simulink model "ROSFeedBackExample"  (R2019b)
settings: Solver=FixedStepDiscrete  StartTime=0.0  StopTime=Inf  FixedStep=0.02  RelTol=1e-3  EnableMultiTasking=on
values from neighbouring files (symbols this model uses):
  m = size(BW, 1)    [ClusterClean.m]    (also in ClusterFuck.m; dotDetection.m)
  X = (round((Ball{1,2}-571)*pixel2mm,2))    [ClusterClean.m]    (also in ClusterFuck.m = (round((Ball{1,2}-CueX)*pixel2mm+30-6.275,2)); PossibleShots.m = (round((balls{1,2})*pixel2mm,2)-6.71); dotDetection.m = rgb2lab(img))
  Y = (round((Ball{1,3}-41)*pixel2mm,2))    [ClusterClean.m]    (also in ClusterFuck.m = (round((Ball{1,3}-CueY)*pixel2mm+30,2)); PossibleShots.m = (round((balls{1,3})*pixel2mm,2)-6.71))
  Z = 80    [ClusterClean.m]    (also in ClusterFuck.m = 90; PossibleShots.m = 90)
undefined symbols (not defined in the file or in its folder): Angular, awayFromGoalThresh, Linear, loadingStation, logicalMap, objectPos, p, q0, refPos, tDuration, tStart, unloadingStations
libraries: sm_lib x153, nesl_utility x33, robotlib x7, robotmaniplib x5, simulink x3, robotalgslib x1
(part 1 of 4)
settings Model: Creator=The MathWorks, Inc.  LastModifiedBy=ryanl
settings DataIOCC: LimitDataPoints=on  SaveFormat=Array  ReturnWorkspaceOutputs=off
settings OptimizationCC: LifeSpan=Inf  MaxStackSize=64
settings DebuggingCC: SolverPrmCheckMsg=warning  AllowSymbolicDim=off  SFUnexpectedBacktrackingDiag=warning  SFNoUnconditionalDefaultTransitionDiag=warning  SFExecutionAtInitializationDiag=none  ArithmeticOperatorsInVariantConditions=warning
settings HardwareCC: ProdBitPerPointer=32  ProdBitPerSizeT=32  ProdBitPerPtrDiffT=32  ProdLargestAtomicFloat=None  ProdIntDivRoundTo=Undefined  ProdEndianess=Unspecified  ProdWordSize=32  ProdHWDeviceType=Generic->Unspecified (assume 32-bit Generic)  TargetHWDeviceType=Generic->Unspecified (assume 32-bit Generic)  UseEmbeddedCoderFeatures=off
settings ModelReferenceCC: PropagateSignalLabelsOutOfModel=off
settings SFSimCC: SimUseLocalCustomCode=off  CustomCodeUndefinedFunction=UseInterfaceOnly
settings RTWCC: SystemTargetFile=ert.tlc  HardwareBoard=Robot Operating System (ROS)  TemplateMakefile=ert_default_tmf  RTWUseLocalCustomCode=off  Toolchain=Catkin  TargetLang=C++
settings CodeAppCC: StateflowObjectComments=on
settings ERTTargetCC: MultiwordLength=2048  ERTCustomFileBanners=off  MultiInstanceERTCode=on  CodeInterfacePackaging=C++ class  SupportContinuousTime=on  SupportNonInlinedSFcns=on  RemoveResetFunc=off  SupportVariableSizeSignals=on  ModelStepFunctionPrototypeControlCompliant=off  RootIOFormat=Structure reference  ConvertIfToSwitch=off  SuppressUnreachableDefaultCases=off
settings ConfigComp: CovMetricSettings=dw  CovHtmlReporting=on  CovSaveCumulativeToWorkspaceVar=on  CovSaveSingleToWorkspaceVar=on  CovExternalEMLEnable=off  CovSFcnEnable=off

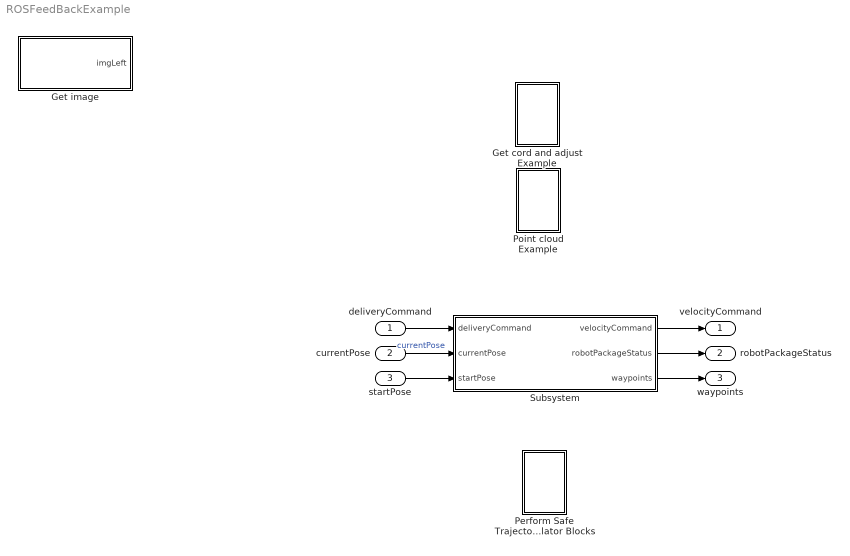
== system ROSFeedBackExample ==
  deliveryCommand : Inport  OutDataTypeStr=Bus: RobotDeliverCommand  BusOutputAsStruct=on
  currentPose : Inport  Port=2  PortDimensions=[3, 1]
  startPose : Inport  Port=3
  Get cord and adjust Example : Subsystem
  Get image : Subsystem
  Perform Safe Trajectory Tracking Control Using Robotics Manipulator Blocks : Subsystem
  Point cloud Example : Subsystem
  Subsystem : Subsystem
  velocityCommand : Outport
  robotPackageStatus : Outport  Port=2  OutDataTypeStr=Bus: RobotPackageStatus  BusOutputAsStruct=on
  waypoints : Outport  Port=3
  wires:
  deliveryCommand/1 -> Subsystem/1(deliveryCommand)
  currentPose/1 -> Subsystem/2(currentPose)  "currentPose"
  startPose/1 -> Subsystem/3(startPose)
  Subsystem/1(velocityCommand) -> velocityCommand/1
  Subsystem/2(robotPackageStatus) -> robotPackageStatus/1
  Subsystem/3(waypoints) -> waypoints/1

== system ROSFeedBackExample/Get cord and adjust Example ==
  note: The /odom topic represents orientation as a quarternion, so convert it to a yaw angle
  note: The desired (X,Y) position of the robot
      | (Colored blocks indicate tunable parameters)
  note: Feedback Control of a ROS-enabled Robot
  note: Copyright 2014-2016 The MathWorks, Inc.
  Bus Selector3 : BusSelector  OutputSignals=Pose.Pose.Position.X,Pose.Pose.Position.Y,Pose.Pose.Orientation.X,Pose.Pose.Orientation.Y,Pose.Pose.Orientation.Z,Pose.Pose.Orientation.W
  Command Velocity Publisher : Subsystem
  Conversion : MATLAB Function  TreatAsAtomicUnit=on
  Desired Position : Constant  Value=[-10 10]
  More Info : Subsystem
      settings: OpenFcn=showdemo(bdroot(gcb))
      mask Display: disp('?')
  Proportional Controller : Subsystem
  Scope : Scope
  Simulation Rate Control : MATLABSystem  System=ExampleHelperSimulationRateControl  SampleTime=0.02
      mask Type: ExampleHelperSimulationRateControl
      mask Display: disp('Rate Control');
  Subscribe : robotlib/Subscribe  topicSource=Select from ROS network  topic=/odom  messageType=nav_msgs/Odometry  sampleTime=-1  messageQueueLength=51
      settings: SourceProductName=ROS Toolbox
  wires:
  Bus Selector3/1 -> Proportional Controller/2(Position X)  "<X>"
  Subscribe/2 -> Bus Selector3/1
  Proportional Controller/1(Linear Velocity (v)) -> Command Velocity Publisher/1(v)
  Conversion/1(yaw) -> Proportional Controller/4(Orientation (theta))
  Desired Position/1 -> Proportional Controller/1(Desired position)
  Bus Selector3/2 -> Proportional Controller/3(Position Y)  "<Y>"
  Bus Selector3/3 -> Conversion/1(x)  "<X>"
  Bus Selector3/5 -> Conversion/3(z)  "<Z>"
  Subscribe/1 -> Command Velocity Publisher/Enable, Scope/1, Proportional Controller/Enable  "IsNew"
  Bus Selector3/4 -> Conversion/2(y)  "<Y>"
  Bus Selector3/6 -> Conversion/4(w)  "<W>"
  Proportional Controller/2(Angular Velocity (w)) -> Command Velocity Publisher/2(w)

== system ROSFeedBackExample/Get image ==
  note: Get Image AND Display
  Error Code Output : Display
  New Message : Display
  Read Image : robotlib/Read Image  MaximumImageSize=[480, 640]  ImageEncoding=rgb8  ShowAlphaOutput=off  ShowErrorCodeOutput=on  VariableSizeOutputs=off
      settings: SourceProductName=ROS Toolbox  SourceProductBaseCode=RR
  Video Viewer1 : VideoViewer  FigPos=[515 695 646 522]
  imgLeftSubscriber : robotlib/Subscribe  topicSource=Select from ROS network  topic=/image_test  messageType=sensor_msgs/Image  sampleTime=-1  messageQueueLength=1
      settings: SourceProductName=ROS Toolbox
  imgLeft : Outport
  wires:
  imgLeftSubscriber/2 -> Read Image/1
  Read Image/1 -> imgLeft/1, Video Viewer1/1
  Read Image/2 -> Error Code Output/1
  imgLeftSubscriber/1 -> New Message/1

== system ROSFeedBackExample/Perform Safe Trajectory Tracking Control Using Robotics Manipulator Blocks ==
  note: Slider to adjust the planar object position
  note: Perform Safe Trajectory Tracking Control Using Robotics Manipulator Blocks
  note: Copyright 2017-2018 The MathWorks, Inc.
  note: Switch to toggle
      | trajectory scaling
  Clock : Clock
  Computed Torque Controller : Subsystem
  Simscape Model with Simple Contact Mechanics : Subsystem
  Simulation Rate Control : MATLABSystem  System=ExampleHelperSimulationRateControl  SampleTime=0.005
      mask Type: ExampleHelperSimulationRateControl
      mask Display: disp('Rate Control');
  Slider : SliderBlock  ScaleMin=0.40000000000000002  ScaleMax=0.80000000000000004
  Toggle Switch : ToggleSwitchBlock  LabelPosition=Hide
      settings: Values={{'Off', 'On'}, [0 1]}
  Trajectory Scaling and Desired Motion : Subsystem
  wires:
  Trajectory Scaling and Desired Motion/1(qd) -> Computed Torque Controller/3(qd)
  Simscape Model with Simple Contact Mechanics/3(torque) -> Trajectory Scaling and Desired Motion/2(torque)
  Computed Torque Controller/1(u) -> Simscape Model with Simple Contact Mechanics/1(u)  "Torque Input"
  Trajectory Scaling and Desired Motion/3(ddqd) -> Computed Torque Controller/5(ddqd)
  Clock/1 -> Trajectory Scaling and Desired Motion/1(clock)
  Trajectory Scaling and Desired Motion/2(dqd) -> Computed Torque Controller/4(dqd)
  Simscape Model with Simple Contact Mechanics/2(dq) -> Computed Torque Controller/2(dq)
  Simscape Model with Simple Contact Mechanics/1(q) -> Computed Torque Controller/1(q)

== system ROSFeedBackExample/Point cloud Example ==
  note: Copyright 2018 The MathWorks, Inc.
  Error Code Output : Display
  MATLAB Function : MATLAB Function  TreatAsAtomicUnit=on
  New Message : Display
  Read Point Cloud : robotlib/Read Point Cloud  MaximumPointCloudSize=[480, 640]  PreserveStructure=on  ShowRGBOutput=on  ShowIntensityOutput=off  ShowErrorCodeOutput=on  VariableSizeOutputs=off
      settings: SourceProductName=ROS Toolbox  SourceProductBaseCode=RR
  Subscribe : robotlib/Subscribe  topicSource=Select from ROS network  topic=/ptcloud_test  messageType=sensor_msgs/PointCloud2  sampleTime=-1  messageQueueLength=1
      settings: SourceProductName=ROS Toolbox
  Video Viewer : VideoViewer  FigPos=[221 634 782 416]
  XYZ Center of Mass : Display
  wires:
  MATLAB Function/1(comXYZ) -> XYZ Center of Mass/1
  Subscribe/1 -> New Message/1
  Read Point Cloud/2 -> Video Viewer/1
  Read Point Cloud/3 -> Error Code Output/1
  Read Point Cloud/1 -> MATLAB Function/1(xyzPoints)
  Subscribe/2 -> Read Point Cloud/1

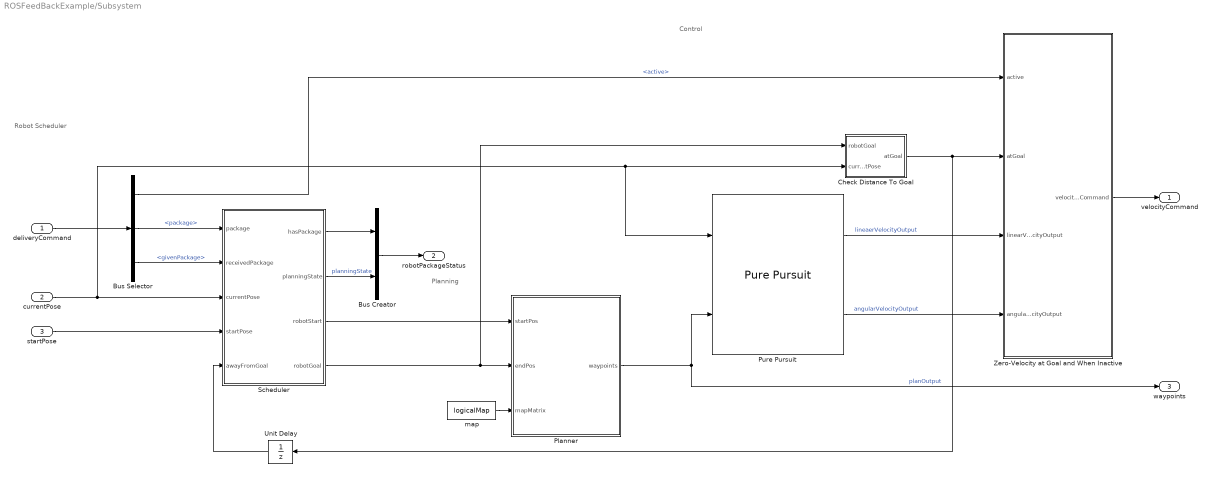
== system ROSFeedBackExample/Subsystem ==
  note: Control
  note: Planning
  note: Robot Scheduler
  deliveryCommand : Inport  OutDataTypeStr=Bus: RobotDeliverCommand  BusOutputAsStruct=on
  currentPose : Inport  Port=2  PortDimensions=[3, 1]
  startPose : Inport  Port=3
  Bus Creator : BusCreator  Inputs=2  OutDataTypeStr=Bus: RobotPackageStatus  NonVirtualBus=on
      settings: InheritFromInputs=off
  Bus Selector : BusSelector  OutputSignals=active,package,givenPackage
  Check Distance To Goal : Subsystem
  Planner : MATLAB Function  TreatAsAtomicUnit=on
  Pure Pursuit : robotalgslib/Pure Pursuit  DesiredLinearVelocity=0.1  MaxAngularVelocity=1.0  LookaheadDistance=0.5  TargetDirPort=off  SimulateUsing=Code generation
      settings: SourceProductName=Navigation Toolbox  SourceProductBaseCode=NV
  Scheduler : Stateflow chart  Priority=2  BlockKeywords=__PRM__SERIALIZED__DATA__:Stateflow Chart,Stateflow Diagram
  Unit Delay : UnitDelay  SampleTime=-1  HasFrameUpgradeWarning=on
  Zero-Velocity at Goal and When Inactive : Subsystem
  map : Constant  Value=logicalMap
  velocityCommand : Outport
  robotPackageStatus : Outport  Port=2  OutDataTypeStr=Bus: RobotPackageStatus  BusOutputAsStruct=on
  waypoints : Outport  Port=3
  wires:
  Pure Pursuit/2 -> Zero-Velocity at Goal and When Inactive/4(angularVelocityOutput)  "angularVelocityOutput"
  map/1 -> Planner/3(mapMatrix)
  Scheduler/1(hasPackage) -> Bus Creator/1
  Bus Selector/1 -> Zero-Velocity at Goal and When Inactive/1(active)  "<active>"
  Unit Delay/1 -> Scheduler/5(awayFromGoal)
  Zero-Velocity at Goal and When Inactive/1(velocityCommand) -> velocityCommand/1
  Planner/1(waypoints) -> waypoints/1, Pure Pursuit/2  "planOutput"
  Pure Pursuit/1 -> Zero-Velocity at Goal and When Inactive/3(linearVelocityOutput)  "lineaerVelocityOutput"
  deliveryCommand/1 -> Bus Selector/1
  Bus Selector/2 -> Scheduler/1(package)  "<package>"
  Scheduler/3(robotStart) -> Planner/1(startPos)
  startPose/1 -> Scheduler/4(startPose)
  Bus Creator/1 -> robotPackageStatus/1
  currentPose/1 -> Pure Pursuit/1, Check Distance To Goal/2(currentPose), Scheduler/3(currentPose)
  Check Distance To Goal/1(atGoal) -> Unit Delay/1, Zero-Velocity at Goal and When Inactive/2(atGoal)
  Scheduler/4(robotGoal) -> Planner/2(endPos), Check Distance To Goal/1(robotGoal)
  Bus Selector/3 -> Scheduler/2(receivedPackage)  "<givenPackage>"
  Scheduler/2(planningState) -> Bus Creator/2  "planningState"

== system ROSFeedBackExample/Get cord and adjust Example/Command Velocity Publisher ==
  v : Inport
  w : Inport  Port=2
  Enable : EnablePort
  Blank Message : robotlib/Blank Message  messageClass=Message  entityType=geometry_msgs/Twist  messageType=geometry_msgs/Twist  SampleTime=inf
      settings: SourceProductName=ROS Toolbox
  Bus Assignment1 : BusAssignment  DialogController=Simulink.DDGSource_BusAssignment  AssignedSignals=Linear.X,Angular.Z
  Publish2 : robotlib/Publish  topicSource=Select from ROS network  topic=/mobile_base/commands/velocity  messageType=geometry_msgs/Twist  messageQueueLength=105
      settings: SourceProductName=ROS Toolbox
  wires:
  Bus Assignment1/1 -> Publish2/1
  Blank Message/1 -> Bus Assignment1/1
  v/1 -> Bus Assignment1/2
  w/1 -> Bus Assignment1/3

== system ROSFeedBackExample/Get cord and adjust Example/More Info ==

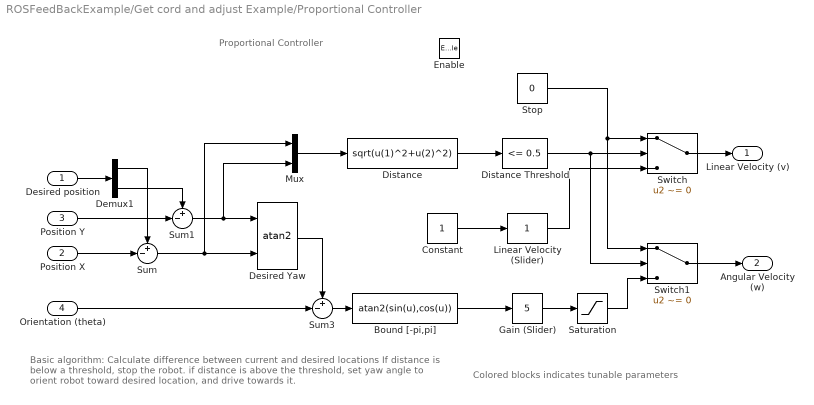
== system ROSFeedBackExample/Get cord and adjust Example/Proportional Controller ==
  note: Proportional Controller
  note: Basic algorithm:
      | Calculate difference between current and desired locations
      | If distance is below a threshold, stop the robot.
      | if distance is above the threshold, set yaw angle to orient robot toward desired location, and drive towards it.
  note: Colored blocks indicates tunable parameters
  Desired position : Inport
  Position X : Inport  Port=2
  Position Y : Inport  Port=3
  Orientation (theta) : Inport  Port=4
  Enable : EnablePort
  Bound [-pi,pi] : Fcn  Expr=atan2(sin(u),cos(u))
  Constant : Constant
  Demux1 : Demux  Outputs=2
  Desired Yaw : Trigonometry  Operator=atan2
  Distance : Fcn  Expr=sqrt(u(1)^2+u(2)^2)
  Distance Threshold : simulink/Logic and Bit Operations/Compare To Constant  relop=<=  const=0.5  OutDataTypeStr=boolean
  Gain (Slider) : simulink/Math Operations/Slider Gain  gain=5  low=1  high=10
  Linear Velocity (Slider) : simulink/Math Operations/Slider Gain  gain=1  low=0  high=2
  Mux : Mux  Inputs=2
  Saturation : Saturate
  Stop : Constant  Value=0
  Sum : Sum  Inputs=+-|
  Sum1 : Sum  Inputs=+-|
  Sum3 : Sum  Inputs=+-|
  Switch : Switch  Criteria=u2 ~= 0
  Switch1 : Switch  Criteria=u2 ~= 0
  Linear Velocity (v) : Outport  VectorParamsAs1DForOutWhenUnconnected=off
  Angular Velocity (w) : Outport  Port=2  VectorParamsAs1DForOutWhenUnconnected=off
  wires:
  Demux1/1 -> Sum/1
  Demux1/2 -> Sum1/1
  Sum1/1 -> Desired Yaw/1, Mux/2
  Constant/1 -> Linear Velocity (Slider)/1
  Desired position/1 -> Demux1/1
  Position Y/1 -> Sum1/2
  Position X/1 -> Sum/2
  Distance/1 -> Distance Threshold/1
  Mux/1 -> Distance/1
  Bound [-pi,pi]/1 -> Gain (Slider)/1
  Orientation (theta)/1 -> Sum3/2
  Desired Yaw/1 -> Sum3/1
  Sum/1 -> Desired Yaw/2, Mux/1
  Distance Threshold/1 -> Switch/2, Switch1/2
  Gain (Slider)/1 -> Saturation/1
  Saturation/1 -> Switch1/3
  Stop/1 -> Switch/1, Switch1/1
  Sum3/1 -> Bound [-pi,pi]/1
  Switch/1 -> Linear Velocity (v)/1
  Linear Velocity (Slider)/1 -> Switch/3
  Switch1/1 -> Angular Velocity (w)/1

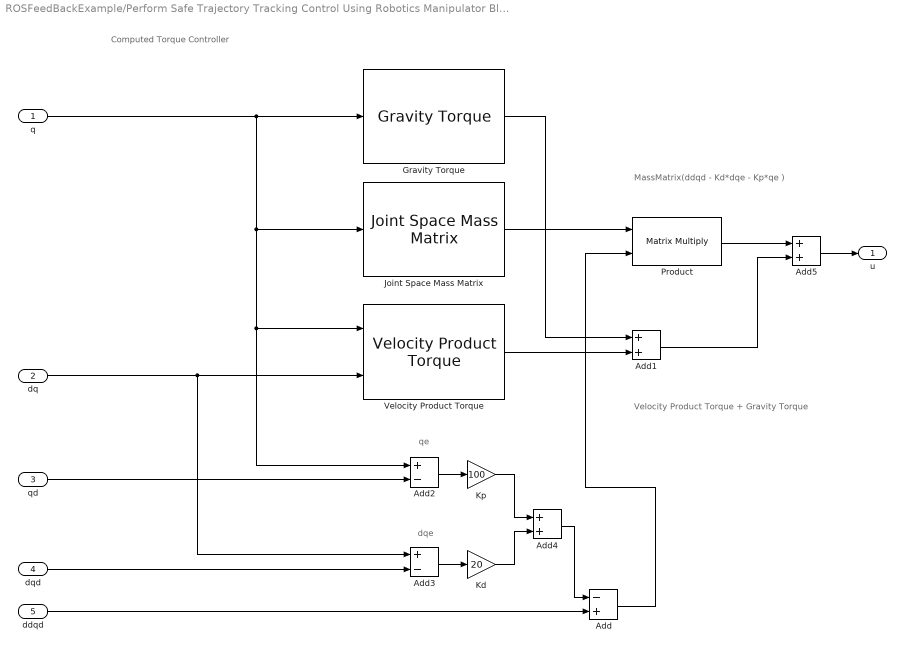
== system ROSFeedBackExample/Perform Safe Trajectory Tracking Control Using Robotics Manipulator Blocks/Computed Torque Controller ==
  note: qe
  note: dqe
  note: Velocity Product Torque + Gravity Torque
  note: MassMatrix(ddqd - Kd*dqe - Kp*qe )
  note: Computed Torque Controller
  q : Inport
  dq : Inport  Port=2
  qd : Inport  Port=3
  dqd : Inport  Port=4
  ddqd : Inport  Port=5
  Add : Sum  Inputs=-+
  Add1 : Sum
  Add2 : Sum  Inputs=+-
  Add3 : Sum  Inputs=+-
  Add4 : Sum
  Add5 : Sum
  Gravity Torque : robotmaniplib/Gravity Torque  RigidBodyTree=sawyer  SimulateUsing=Interpreted execution
      settings: SourceProductName=Robotics System Toolbox
  Joint Space Mass Matrix : robotmaniplib/Joint Space Mass Matrix  RigidBodyTree=sawyer  SimulateUsing=Interpreted execution
      settings: SourceProductName=Robotics System Toolbox
  Kd : Gain  Gain=20
  Kp : Gain  Gain=100
  Product : Product  Multiplication=Matrix(*)
  Velocity Product Torque : robotmaniplib/Velocity Product Torque  RigidBodyTree=sawyer  SimulateUsing=Interpreted execution
      settings: SourceProductName=Robotics System Toolbox  SourceProductBaseCode=RO
  u : Outport  VectorParamsAs1DForOutWhenUnconnected=off
  wires:
  Joint Space Mass Matrix/1 -> Product/1
  q/1 -> Gravity Torque/1, Joint Space Mass Matrix/1, Add2/1, Velocity Product Torque/1
  dq/1 -> Velocity Product Torque/2, Add3/1
  Add4/1 -> Add/1
  ddqd/1 -> Add/2
  Add/1 -> Product/2
  qd/1 -> Add2/2
  dqd/1 -> Add3/2
  Add2/1 -> Kp/1
  Add3/1 -> Kd/1
  Kp/1 -> Add4/1
  Kd/1 -> Add4/2
  Add5/1 -> u/1
  Product/1 -> Add5/1
  Add1/1 -> Add5/2
  Gravity Torque/1 -> Add1/1
  Velocity Product Torque/1 -> Add1/2

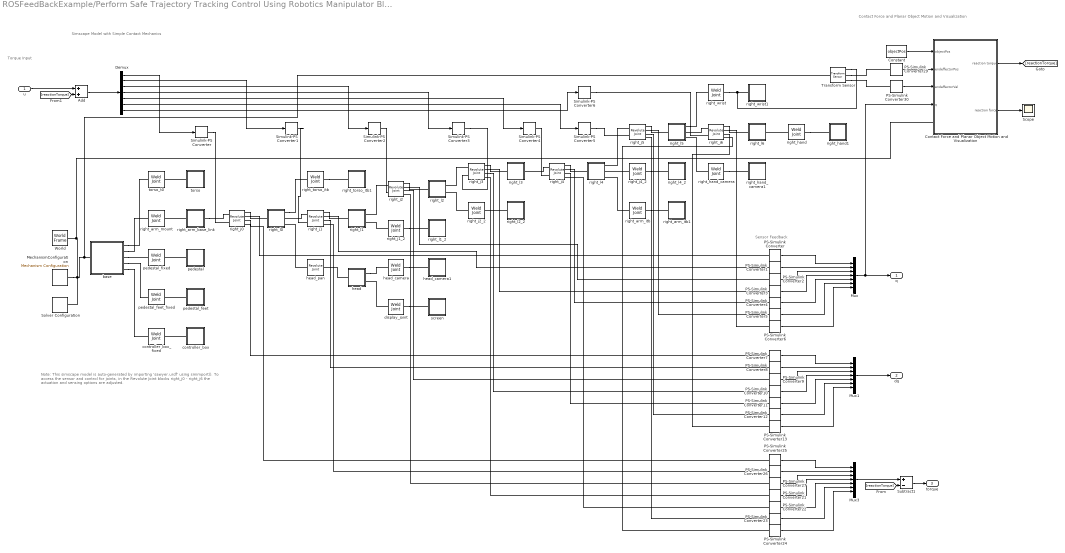
== system ROSFeedBackExample/Perform Safe Trajectory Tracking Control Using Robotics Manipulator Blocks/Simscape Model with Simple Contact Mechanics ==
  note: Contact Force and Planar Object Motion and Visualization
  note: Sensor Feedback
  note: Torque Input
  note: Simscape Model with Simple Contact Mechanics
  note: Note: This simscape model is auto-generated by importing 'sawyer.urdf' using smimport().
      | To access the sensor and control for joints, in the Revolute Joint blocks right_j0 - right_j6
      | the actuation and sensing options are adjusted.
  u : Inport
  Add : Sum
  Constant : Constant  Value=objectPos
  Contact Force and Planar Object Motion and Visualization : Subsystem
  Demux : Demux  Outputs=7
  MechanismConfiguration : sm_lib/Utilities/Mechanism Configuration  UniformGravity=Constant  GravityVector=[0 0 -9.80665]  GravityUnits=m/s^2  LinearizationDelta=0.001
  Mux : Mux  Inputs=7
  Mux1 : Mux  Inputs=7
  Mux3 : Mux  Inputs=7
  PS-Simulink Converter{,1..13,21..27,29..30} (23 alike) : nesl_utility/PS-Simulink Converter  PhysicalDomain=network_engine_domain  SubClassName=ps_output  LeftPortType=input  RightPortType=output  PseudoPeriodic=off  Frequencies=[]  Unit=1  AffineConversion=off
  Scope : Scope
  Simulink-PS Converter{,1..6} (7 alike) : nesl_utility/Simulink-PS Converter  PhysicalDomain=network_engine_domain  SubClassName=ps_input  LeftPortType=input  RightPortType=output  PseudoPeriodic=off  Frequencies=[]  NoiseDistribution=none  NoiseParameters=[]  Unit=1  AffineConversion=off  FilteringAndDerivatives=provide  SimscapeFilterOrder=1  InputFilterTimeConstant=0.001  UdotUserProvided=0
  Solver Configuration : nesl_utility/Solver Configuration  PhysicalDomain=network_engine_domain  SubClassName=solver  LeftPortType=input  RightPortType=generic  Tones=[]  Harmonics=[]  SimulateNoise=off  Profile=off  UseLocalSampling=off  EnableSwitchedLinearOptims=on  FrequencyDomain=off  UseCCode=off  RelTol=0.001  AbsTol=1e-06  MinStep=1e-09  ToWorkspace=off  RevertToSquareIcSolve=off  NumHomotopyIterations=100  PhasorMode=off  PhasorModeNumHarmonics=1  DoDC=off  ResidualTolerance=1e-09  UseLocalSolver=off  LocalSolverChoice=NE_BACKWARD_EULER_ADVANCER  LocalSolverSampleTime=0.001  DoFixedCost=off  MaxNonlinIter=3  MaxModeIter=2  LinearAlgebra=Sparse  EquationFormulation=NE_TIME_EF  DelaysMemoryBudget=1024  AutomaticFiltering=on  FilteringTimeConstant=0.001  PartitionStorageMethod=AS_NEEDED  PartitionMemoryBudget=1024  PartitionMethod=FAST
  Subtract1 : Sum  Inputs=+-
  Transform Sensor : sm_lib/Frames and Transforms/Transform Sensor  MeasurementFrame=World  SenseAngle=off  SenseAxis=off  SenseAngle1=off  SenseAngle2=off  SenseAngle3=off  SenseQ=off  SenseR=off  SenseOmegaX=off  SenseOmegaY=off  SenseOmegaZ=off  SenseOmega1=off  SenseOmega2=off  SenseOmega3=off  SenseQDot=off  SenseRDot=off  SenseAlphaX=off  SenseAlphaY=off  SenseAlphaZ=off  SenseAlpha1=off  SenseAlpha2=off  SenseAlpha3=off  SenseQDDot=off  SenseRDDot=off  SenseX=on  SenseY=off  SenseZ=off  SenseRad=off  SenseAzim=off  SenseDist=off  SenseInc=off  SenseXDot=on  SenseYDot=off  SenseZDot=off  SenseRadDot=off  SenseAzimDot=off  SenseDistDot=off  SenseIncDot=off  SenseXDDot=off  SenseYDDot=off  SenseZDDot=off  SenseRadDDot=off  SenseAzimDDot=off  SenseDistDDot=off  SenseIncDDot=off
  World : sm_lib/Frames and Transforms/World Frame
  base : Subsystem
  controller_box : Subsystem
  controller_box_fixed : sm_lib/Joints/Weld Joint  JointMode=Normal  SenseConstraintForce=off  SenseConstraintForceX=off  SenseConstraintForceY=off  SenseConstraintForceZ=off  SenseConstraintTorque=off  SenseConstraintTorqueX=off  SenseConstraintTorqueY=off  SenseConstraintTorqueZ=off  SenseTotalForce=off  SenseTotalForceX=off  SenseTotalForceY=off  SenseTotalForceZ=off  SenseTotalTorque=off  SenseTotalTorqueX=off  SenseTotalTorqueY=off  SenseTotalTorqueZ=off  CompositeWrenchDir=FollowerOnBase  CompositeWrenchFrame=BaseFrame
  display_joint : sm_lib/Joints/Weld Joint  JointMode=Normal  SenseConstraintForce=off  SenseConstraintForceX=off  SenseConstraintForceY=off  SenseConstraintForceZ=off  SenseConstraintTorque=off  SenseConstraintTorqueX=off  SenseConstraintTorqueY=off  SenseConstraintTorqueZ=off  SenseTotalForce=off  SenseTotalForceX=off  SenseTotalForceY=off  SenseTotalForceZ=off  SenseTotalTorque=off  SenseTotalTorqueX=off  SenseTotalTorqueY=off  SenseTotalTorqueZ=off  CompositeWrenchDir=FollowerOnBase  CompositeWrenchFrame=BaseFrame
  head : Subsystem
  head_camera : sm_lib/Joints/Weld Joint  JointMode=Normal  SenseConstraintForce=off  SenseConstraintForceX=off  SenseConstraintForceY=off  SenseConstraintForceZ=off  SenseConstraintTorque=off  SenseConstraintTorqueX=off  SenseConstraintTorqueY=off  SenseConstraintTorqueZ=off  SenseTotalForce=off  SenseTotalForceX=off  SenseTotalForceY=off  SenseTotalForceZ=off  SenseTotalTorque=off  SenseTotalTorqueX=off  SenseTotalTorqueY=off  SenseTotalTorqueZ=off  CompositeWrenchDir=FollowerOnBase  CompositeWrenchFrame=BaseFrame
  head_camera1 : Subsystem
  head_pan : sm_lib/Joints/Revolute Joint  JointMode=Normal  SenseConstraintForce=off  SenseConstraintForceX=off  SenseConstraintForceY=off  SenseConstraintForceZ=off  SenseConstraintTorque=off  SenseConstraintTorqueX=off  SenseConstraintTorqueY=off  SenseConstraintTorqueZ=off  SenseTotalForce=off  SenseTotalForceX=off  SenseTotalForceY=off  SenseTotalForceZ=off  SenseTotalTorque=off  SenseTotalTorqueX=off  SenseTotalTorqueY=off  SenseTotalTorqueZ=off  CompositeWrenchDir=FollowerOnBase  CompositeWrenchFrame=BaseFrame  EquilibriumPosition=0  EquilibriumPositionUnits=deg  SpringStiffness=0  SpringStiffnessUnits=N*m/deg  DampingCoefficient=0  DampingCoefficientUnits=m^2*kg/s/rad  TorqueActuationMode=NoTorque  MotionActuationMode=ComputedMotion  SensePosition=off  SenseVelocity=off  SenseAcceleration=off  SenseTorqueForce=off  SenseLowerLimitTorqueForce=off  SenseUpperLimitTorqueForce=off  LowerLimitSpecify=off  LowerLimitBound=-90  LowerLimitBoundUnits=deg  LowerLimitStiffness=1e4  LowerLimitStiffnessUnits=N*m/deg  LowerLimitDamping=10  LowerLimitDampingUnits=N*m/(deg/s)  LowerLimitTransitionRegionWidth=0.1  LowerLimitTransitionRegionWidthUnits=deg  UpperLimitSpecify=off  UpperLimitBound=90  UpperLimitBoundUnits=deg  UpperLimitStiffness=1e4  UpperLimitStiffnessUnits=N*m/deg  UpperLimitDamping=10  UpperLimitDampingUnits=N*m/(deg/s)  UpperLimitTransitionRegionWidth=0.1  UpperLimitTransitionRegionWidthUnits=deg  PositionTargetSpecify=off  PositionTargetPriority=High  PositionTargetValue=0  PositionTargetValueUnits=deg  VelocityTargetSpecify=off  VelocityTargetPriority=High  VelocityTargetValue=0  VelocityTargetValueUnits=deg/s
  pedestal : Subsystem
  pedestal_feet : Subsystem
  pedestal_feet_fixed : sm_lib/Joints/Weld Joint  JointMode=Normal  SenseConstraintForce=off  SenseConstraintForceX=off  SenseConstraintForceY=off  SenseConstraintForceZ=off  SenseConstraintTorque=off  SenseConstraintTorqueX=off  SenseConstraintTorqueY=off  SenseConstraintTorqueZ=off  SenseTotalForce=off  SenseTotalForceX=off  SenseTotalForceY=off  SenseTotalForceZ=off  SenseTotalTorque=off  SenseTotalTorqueX=off  SenseTotalTorqueY=off  SenseTotalTorqueZ=off  CompositeWrenchDir=FollowerOnBase  CompositeWrenchFrame=BaseFrame
  pedestal_fixed : sm_lib/Joints/Weld Joint  JointMode=Normal  SenseConstraintForce=off  SenseConstraintForceX=off  SenseConstraintForceY=off  SenseConstraintForceZ=off  SenseConstraintTorque=off  SenseConstraintTorqueX=off  SenseConstraintTorqueY=off  SenseConstraintTorqueZ=off  SenseTotalForce=off  SenseTotalForceX=off  SenseTotalForceY=off  SenseTotalForceZ=off  SenseTotalTorque=off  SenseTotalTorqueX=off  SenseTotalTorqueY=off  SenseTotalTorqueZ=off  CompositeWrenchDir=FollowerOnBase  CompositeWrenchFrame=BaseFrame
  right_arm_base_link : Subsystem
  right_arm_itb : sm_lib/Joints/Weld Joint  JointMode=Normal  SenseConstraintForce=off  SenseConstraintForceX=off  SenseConstraintForceY=off  SenseConstraintForceZ=off  SenseConstraintTorque=off  SenseConstraintTorqueX=off  SenseConstraintTorqueY=off  SenseConstraintTorqueZ=off  SenseTotalForce=off  SenseTotalForceX=off  SenseTotalForceY=off  SenseTotalForceZ=off  SenseTotalTorque=off  SenseTotalTorqueX=off  SenseTotalTorqueY=off  SenseTotalTorqueZ=off  CompositeWrenchDir=FollowerOnBase  CompositeWrenchFrame=BaseFrame
  right_arm_itb1 : Subsystem
  right_arm_mount : sm_lib/Joints/Weld Joint  JointMode=Normal  SenseConstraintForce=off  SenseConstraintForceX=off  SenseConstraintForceY=off  SenseConstraintForceZ=off  SenseConstraintTorque=off  SenseConstraintTorqueX=off  SenseConstraintTorqueY=off  SenseConstraintTorqueZ=off  SenseTotalForce=off  SenseTotalForceX=off  SenseTotalForceY=off  SenseTotalForceZ=off  SenseTotalTorque=off  SenseTotalTorqueX=off  SenseTotalTorqueY=off  SenseTotalTorqueZ=off  CompositeWrenchDir=FollowerOnBase  CompositeWrenchFrame=BaseFrame
  right_hand : sm_lib/Joints/Weld Joint  JointMode=Normal  SenseConstraintForce=off  SenseConstraintForceX=off  SenseConstraintForceY=off  SenseConstraintForceZ=off  SenseConstraintTorque=off  SenseConstraintTorqueX=off  SenseConstraintTorqueY=off  SenseConstraintTorqueZ=off  SenseTotalForce=off  SenseTotalForceX=off  SenseTotalForceY=off  SenseTotalForceZ=off  SenseTotalTorque=off  SenseTotalTorqueX=off  SenseTotalTorqueY=off  SenseTotalTorqueZ=off  CompositeWrenchDir=FollowerOnBase  CompositeWrenchFrame=BaseFrame
  right_hand1 : Subsystem
  right_hand_camera : sm_lib/Joints/Weld Joint  JointMode=Normal  SenseConstraintForce=off  SenseConstraintForceX=off  SenseConstraintForceY=off  SenseConstraintForceZ=off  SenseConstraintTorque=off  SenseConstraintTorqueX=off  SenseConstraintTorqueY=off  SenseConstraintTorqueZ=off  SenseTotalForce=off  SenseTotalForceX=off  SenseTotalForceY=off  SenseTotalForceZ=off  SenseTotalTorque=off  SenseTotalTorqueX=off  SenseTotalTorqueY=off  SenseTotalTorqueZ=off  CompositeWrenchDir=FollowerOnBase  CompositeWrenchFrame=BaseFrame
  right_hand_camera1 : Subsystem
  right_j0 : sm_lib/Joints/Revolute Joint  JointMode=Normal  SenseConstraintForce=off  SenseConstraintForceX=off  SenseConstraintForceY=off  SenseConstraintForceZ=off  SenseConstraintTorque=off  SenseConstraintTorqueX=off  SenseConstraintTorqueY=off  SenseConstraintTorqueZ=off  SenseTotalForce=off  SenseTotalForceX=off  SenseTotalForceY=off  SenseTotalForceZ=off  SenseTotalTorque=off  SenseTotalTorqueX=off  SenseTotalTorqueY=off  SenseTotalTorqueZ=off  CompositeWrenchDir=FollowerOnBase  CompositeWrenchFrame=BaseFrame  EquilibriumPosition=0  EquilibriumPositionUnits=deg  SpringStiffness=0  SpringStiffnessUnits=N*m/deg  DampingCoefficient=0  DampingCoefficientUnits=m^2*kg/s/rad  TorqueActuationMode=InputTorque  MotionActuationMode=ComputedMotion  SensePosition=on  SenseVelocity=on  SenseAcceleration=off  SenseTorqueForce=on  SenseLowerLimitTorqueForce=off  SenseUpperLimitTorqueForce=off  LowerLimitSpecify=off  LowerLimitBound=-90  LowerLimitBoundUnits=deg  LowerLimitStiffness=1e4  LowerLimitStiffnessUnits=N*m/deg  LowerLimitDamping=10  LowerLimitDampingUnits=N*m/(deg/s)  LowerLimitTransitionRegionWidth=0.1  LowerLimitTransitionRegionWidthUnits=deg  UpperLimitSpecify=off  UpperLimitBound=90  UpperLimitBoundUnits=deg  UpperLimitStiffness=1e4  UpperLimitStiffnessUnits=N*m/deg  UpperLimitDamping=10  UpperLimitDampingUnits=N*m/(deg/s)  UpperLimitTransitionRegionWidth=0.1  UpperLimitTransitionRegionWidthUnits=deg  PositionTargetSpecify=on  PositionTargetPriority=High  PositionTargetValue=q0(1)  PositionTargetValueUnits=rad  VelocityTargetSpecify=off  VelocityTargetPriority=High  VelocityTargetValue=0  VelocityTargetValueUnits=deg/s
  right_j1 : sm_lib/Joints/Revolute Joint  JointMode=Normal  SenseConstraintForce=off  SenseConstraintForceX=off  SenseConstraintForceY=off  SenseConstraintForceZ=off  SenseConstraintTorque=off  SenseConstraintTorqueX=off  SenseConstraintTorqueY=off  SenseConstraintTorqueZ=off  SenseTotalForce=off  SenseTotalForceX=off  SenseTotalForceY=off  SenseTotalForceZ=off  SenseTotalTorque=off  SenseTotalTorqueX=off  SenseTotalTorqueY=off  SenseTotalTorqueZ=off  CompositeWrenchDir=FollowerOnBase  CompositeWrenchFrame=BaseFrame  EquilibriumPosition=0  EquilibriumPositionUnits=deg  SpringStiffness=0  SpringStiffnessUnits=N*m/deg  DampingCoefficient=0  DampingCoefficientUnits=m^2*kg/s/rad  TorqueActuationMode=InputTorque  MotionActuationMode=ComputedMotion  SensePosition=on  SenseVelocity=on  SenseAcceleration=off  SenseTorqueForce=on  SenseLowerLimitTorqueForce=off  SenseUpperLimitTorqueForce=off  LowerLimitSpecify=off  LowerLimitBound=-90  LowerLimitBoundUnits=deg  LowerLimitStiffness=1e4  LowerLimitStiffnessUnits=N*m/deg  LowerLimitDamping=10  LowerLimitDampingUnits=N*m/(deg/s)  LowerLimitTransitionRegionWidth=0.1  LowerLimitTransitionRegionWidthUnits=deg  UpperLimitSpecify=off  UpperLimitBound=90  UpperLimitBoundUnits=deg  UpperLimitStiffness=1e4  UpperLimitStiffnessUnits=N*m/deg  UpperLimitDamping=10  UpperLimitDampingUnits=N*m/(deg/s)  UpperLimitTransitionRegionWidth=0.1  UpperLimitTransitionRegionWidthUnits=deg  PositionTargetSpecify=on  PositionTargetPriority=High  PositionTargetValue=q0(2)  PositionTargetValueUnits=rad  VelocityTargetSpecify=off  VelocityTargetPriority=High  VelocityTargetValue=0  VelocityTargetValueUnits=deg/s
  right_j1_2 : sm_lib/Joints/Weld Joint  JointMode=Normal  SenseConstraintForce=off  SenseConstraintForceX=off  SenseConstraintForceY=off  SenseConstraintForceZ=off  SenseConstraintTorque=off  SenseConstraintTorqueX=off  SenseConstraintTorqueY=off  SenseConstraintTorqueZ=off  SenseTotalForce=off  SenseTotalForceX=off  SenseTotalForceY=off  SenseTotalForceZ=off  SenseTotalTorque=off  SenseTotalTorqueX=off  SenseTotalTorqueY=off  SenseTotalTorqueZ=off  CompositeWrenchDir=FollowerOnBase  CompositeWrenchFrame=BaseFrame
  right_j2 : sm_lib/Joints/Revolute Joint  JointMode=Normal  SenseConstraintForce=off  SenseConstraintForceX=off  SenseConstraintForceY=off  SenseConstraintForceZ=off  SenseConstraintTorque=off  SenseConstraintTorqueX=off  SenseConstraintTorqueY=off  SenseConstraintTorqueZ=off  SenseTotalForce=off  SenseTotalForceX=off  SenseTotalForceY=off  SenseTotalForceZ=off  SenseTotalTorque=off  SenseTotalTorqueX=off  SenseTotalTorqueY=off  SenseTotalTorqueZ=off  CompositeWrenchDir=FollowerOnBase  CompositeWrenchFrame=BaseFrame  EquilibriumPosition=0  EquilibriumPositionUnits=deg  SpringStiffness=0  SpringStiffnessUnits=N*m/deg  DampingCoefficient=0  DampingCoefficientUnits=m^2*kg/s/rad  TorqueActuationMode=InputTorque  MotionActuationMode=ComputedMotion  SensePosition=on  SenseVelocity=on  SenseAcceleration=off  SenseTorqueForce=on  SenseLowerLimitTorqueForce=off  SenseUpperLimitTorqueForce=off  LowerLimitSpecify=off  LowerLimitBound=-90  LowerLimitBoundUnits=deg  LowerLimitStiffness=1e4  LowerLimitStiffnessUnits=N*m/deg  LowerLimitDamping=10  LowerLimitDampingUnits=N*m/(deg/s)  LowerLimitTransitionRegionWidth=0.1  LowerLimitTransitionRegionWidthUnits=deg  UpperLimitSpecify=off  UpperLimitBound=90  UpperLimitBoundUnits=deg  UpperLimitStiffness=1e4  UpperLimitStiffnessUnits=N*m/deg  UpperLimitDamping=10  UpperLimitDampingUnits=N*m/(deg/s)  UpperLimitTransitionRegionWidth=0.1  UpperLimitTransitionRegionWidthUnits=deg  PositionTargetSpecify=on  PositionTargetPriority=High  PositionTargetValue=q0(3)  PositionTargetValueUnits=rad  VelocityTargetSpecify=off  VelocityTargetPriority=High  VelocityTargetValue=0  VelocityTargetValueUnits=deg/s
  right_j2_2 : sm_lib/Joints/Weld Joint  JointMode=Normal  SenseConstraintForce=off  SenseConstraintForceX=off  SenseConstraintForceY=off  SenseConstraintForceZ=off  SenseConstraintTorque=off  SenseConstraintTorqueX=off  SenseConstraintTorqueY=off  SenseConstraintTorqueZ=off  SenseTotalForce=off  SenseTotalForceX=off  SenseTotalForceY=off  SenseTotalForceZ=off  SenseTotalTorque=off  SenseTotalTorqueX=off  SenseTotalTorqueY=off  SenseTotalTorqueZ=off  CompositeWrenchDir=FollowerOnBase  CompositeWrenchFrame=BaseFrame
  right_j3 : sm_lib/Joints/Revolute Joint  JointMode=Normal  SenseConstraintForce=off  SenseConstraintForceX=off  SenseConstraintForceY=off  SenseConstraintForceZ=off  SenseConstraintTorque=off  SenseConstraintTorqueX=off  SenseConstraintTorqueY=off  SenseConstraintTorqueZ=off  SenseTotalForce=off  SenseTotalForceX=off  SenseTotalForceY=off  SenseTotalForceZ=off  SenseTotalTorque=off  SenseTotalTorqueX=off  SenseTotalTorqueY=off  SenseTotalTorqueZ=off  CompositeWrenchDir=FollowerOnBase  CompositeWrenchFrame=BaseFrame  EquilibriumPosition=0  EquilibriumPositionUnits=deg  SpringStiffness=0  SpringStiffnessUnits=N*m/deg  DampingCoefficient=0  DampingCoefficientUnits=m^2*kg/s/rad  TorqueActuationMode=InputTorque  MotionActuationMode=ComputedMotion  SensePosition=on  SenseVelocity=on  SenseAcceleration=off  SenseTorqueForce=on  SenseLowerLimitTorqueForce=off  SenseUpperLimitTorqueForce=off  LowerLimitSpecify=off  LowerLimitBound=-90  LowerLimitBoundUnits=deg  LowerLimitStiffness=1e4  LowerLimitStiffnessUnits=N*m/deg  LowerLimitDamping=10  LowerLimitDampingUnits=N*m/(deg/s)  LowerLimitTransitionRegionWidth=0.1  LowerLimitTransitionRegionWidthUnits=deg  UpperLimitSpecify=off  UpperLimitBound=90  UpperLimitBoundUnits=deg  UpperLimitStiffness=1e4  UpperLimitStiffnessUnits=N*m/deg  UpperLimitDamping=10  UpperLimitDampingUnits=N*m/(deg/s)  UpperLimitTransitionRegionWidth=0.1  UpperLimitTransitionRegionWidthUnits=deg  PositionTargetSpecify=on  PositionTargetPriority=High  PositionTargetValue=q0(4)  PositionTargetValueUnits=rad  VelocityTargetSpecify=off  VelocityTargetPriority=High  VelocityTargetValue=0  VelocityTargetValueUnits=deg/s
  right_j4 : sm_lib/Joints/Revolute Joint  JointMode=Normal  SenseConstraintForce=off  SenseConstraintForceX=off  SenseConstraintForceY=off  SenseConstraintForceZ=off  SenseConstraintTorque=off  SenseConstraintTorqueX=off  SenseConstraintTorqueY=off  SenseConstraintTorqueZ=off  SenseTotalForce=off  SenseTotalForceX=off  SenseTotalForceY=off  SenseTotalForceZ=off  SenseTotalTorque=off  SenseTotalTorqueX=off  SenseTotalTorqueY=off  SenseTotalTorqueZ=off  CompositeWrenchDir=FollowerOnBase  CompositeWrenchFrame=BaseFrame  EquilibriumPosition=0  EquilibriumPositionUnits=deg  SpringStiffness=0  SpringStiffnessUnits=N*m/deg  DampingCoefficient=0  DampingCoefficientUnits=m^2*kg/s/rad  TorqueActuationMode=InputTorque  MotionActuationMode=ComputedMotion  SensePosition=on  SenseVelocity=on  SenseAcceleration=off  SenseTorqueForce=on  SenseLowerLimitTorqueForce=off  SenseUpperLimitTorqueForce=off  LowerLimitSpecify=off  LowerLimitBound=-90  LowerLimitBoundUnits=deg  LowerLimitStiffness=1e4  LowerLimitStiffnessUnits=N*m/deg  LowerLimitDamping=10  LowerLimitDampingUnits=N*m/(deg/s)  LowerLimitTransitionRegionWidth=0.1  LowerLimitTransitionRegionWidthUnits=deg  UpperLimitSpecify=off  UpperLimitBound=90  UpperLimitBoundUnits=deg  UpperLimitStiffness=1e4  UpperLimitStiffnessUnits=N*m/deg  UpperLimitDamping=10  UpperLimitDampingUnits=N*m/(deg/s)  UpperLimitTransitionRegionWidth=0.1  UpperLimitTransitionRegionWidthUnits=deg  PositionTargetSpecify=on  PositionTargetPriority=High  PositionTargetValue=q0(5)  PositionTargetValueUnits=rad  VelocityTargetSpecify=off  VelocityTargetPriority=High  VelocityTargetValue=0  VelocityTargetValueUnits=deg/s
  right_j4_2 : sm_lib/Joints/Weld Joint  JointMode=Normal  SenseConstraintForce=off  SenseConstraintForceX=off  SenseConstraintForceY=off  SenseConstraintForceZ=off  SenseConstraintTorque=off  SenseConstraintTorqueX=off  SenseConstraintTorqueY=off  SenseConstraintTorqueZ=off  SenseTotalForce=off  SenseTotalForceX=off  SenseTotalForceY=off  SenseTotalForceZ=off  SenseTotalTorque=off  SenseTotalTorqueX=off  SenseTotalTorqueY=off  SenseTotalTorqueZ=off  CompositeWrenchDir=FollowerOnBase  CompositeWrenchFrame=BaseFrame
  right_j5 : sm_lib/Joints/Revolute Joint  JointMode=Normal  SenseConstraintForce=off  SenseConstraintForceX=off  SenseConstraintForceY=off  SenseConstraintForceZ=off  SenseConstraintTorque=off  SenseConstraintTorqueX=off  SenseConstraintTorqueY=off  SenseConstraintTorqueZ=off  SenseTotalForce=off  SenseTotalForceX=off  SenseTotalForceY=off  SenseTotalForceZ=off  SenseTotalTorque=off  SenseTotalTorqueX=off  SenseTotalTorqueY=off  SenseTotalTorqueZ=off  CompositeWrenchDir=FollowerOnBase  CompositeWrenchFrame=BaseFrame  EquilibriumPosition=0  EquilibriumPositionUnits=deg  SpringStiffness=0  SpringStiffnessUnits=N*m/deg  DampingCoefficient=0  DampingCoefficientUnits=m^2*kg/s/rad  TorqueActuationMode=InputTorque  MotionActuationMode=ComputedMotion  SensePosition=on  SenseVelocity=on  SenseAcceleration=off  SenseTorqueForce=on  SenseLowerLimitTorqueForce=off  SenseUpperLimitTorqueForce=off  LowerLimitSpecify=off  LowerLimitBound=-90  LowerLimitBoundUnits=deg  LowerLimitStiffness=1e4  LowerLimitStiffnessUnits=N*m/deg  LowerLimitDamping=10  LowerLimitDampingUnits=N*m/(deg/s)  LowerLimitTransitionRegionWidth=0.1  LowerLimitTransitionRegionWidthUnits=deg  UpperLimitSpecify=off  UpperLimitBound=90  UpperLimitBoundUnits=deg  UpperLimitStiffness=1e4  UpperLimitStiffnessUnits=N*m/deg  UpperLimitDamping=10  UpperLimitDampingUnits=N*m/(deg/s)  UpperLimitTransitionRegionWidth=0.1  UpperLimitTransitionRegionWidthUnits=deg  PositionTargetSpecify=on  PositionTargetPriority=High  PositionTargetValue=q0(6)  PositionTargetValueUnits=rad  VelocityTargetSpecify=off  VelocityTargetPriority=High  VelocityTargetValue=0  VelocityTargetValueUnits=deg/s
  right_j6 : sm_lib/Joints/Revolute Joint  JointMode=Normal  SenseConstraintForce=off  SenseConstraintForceX=off  SenseConstraintForceY=off  SenseConstraintForceZ=off  SenseConstraintTorque=off  SenseConstraintTorqueX=off  SenseConstraintTorqueY=off  SenseConstraintTorqueZ=off  SenseTotalForce=off  SenseTotalForceX=off  SenseTotalForceY=off  SenseTotalForceZ=off  SenseTotalTorque=off  SenseTotalTorqueX=off  SenseTotalTorqueY=off  SenseTotalTorqueZ=off  CompositeWrenchDir=FollowerOnBase  CompositeWrenchFrame=BaseFrame  EquilibriumPosition=0  EquilibriumPositionUnits=deg  SpringStiffness=0  SpringStiffnessUnits=N*m/deg  DampingCoefficient=0  DampingCoefficientUnits=m^2*kg/s/rad  TorqueActuationMode=InputTorque  MotionActuationMode=ComputedMotion  SensePosition=on  SenseVelocity=on  SenseAcceleration=off  SenseTorqueForce=on  SenseLowerLimitTorqueForce=off  SenseUpperLimitTorqueForce=off  LowerLimitSpecify=off  LowerLimitBound=-90  LowerLimitBoundUnits=deg  LowerLimitStiffness=1e4  LowerLimitStiffnessUnits=N*m/deg  LowerLimitDamping=10  LowerLimitDampingUnits=N*m/(deg/s)  LowerLimitTransitionRegionWidth=0.1  LowerLimitTransitionRegionWidthUnits=deg  UpperLimitSpecify=off  UpperLimitBound=90  UpperLimitBoundUnits=deg  UpperLimitStiffness=1e4  UpperLimitStiffnessUnits=N*m/deg  UpperLimitDamping=10  UpperLimitDampingUnits=N*m/(deg/s)  UpperLimitTransitionRegionWidth=0.1  UpperLimitTransitionRegionWidthUnits=deg  PositionTargetSpecify=on  PositionTargetPriority=High  PositionTargetValue=q0(7)  PositionTargetValueUnits=rad  VelocityTargetSpecify=off  VelocityTargetPriority=High  VelocityTargetValue=0  VelocityTargetValueUnits=deg/s
  right_l0 : Subsystem
  right_l1 : Subsystem
  right_l1_2 : Subsystem
  right_l2 : Subsystem
  right_l2_2 : Subsystem
  right_l3 : Subsystem
  right_l4 : Subsystem
  right_l4_2 : Subsystem
  right_l5 : Subsystem
  right_l6 : Subsystem
  right_torso_itb : sm_lib/Joints/Weld Joint  JointMode=Normal  SenseConstraintForce=off  SenseConstraintForceX=off  SenseConstraintForceY=off  SenseConstraintForceZ=off  SenseConstraintTorque=off  SenseConstraintTorqueX=off  SenseConstraintTorqueY=off  SenseConstraintTorqueZ=off  SenseTotalForce=off  SenseTotalForceX=off  SenseTotalForceY=off  SenseTotalForceZ=off  SenseTotalTorque=off  SenseTotalTorqueX=off  SenseTotalTorqueY=off  SenseTotalTorqueZ=off  CompositeWrenchDir=FollowerOnBase  CompositeWrenchFrame=BaseFrame
  right_torso_itb1 : Subsystem
  right_wrist : sm_lib/Joints/Weld Joint  JointMode=Normal  SenseConstraintForce=off  SenseConstraintForceX=off  SenseConstraintForceY=off  SenseConstraintForceZ=off  SenseConstraintTorque=off  SenseConstraintTorqueX=off  SenseConstraintTorqueY=off  SenseConstraintTorqueZ=off  SenseTotalForce=off  SenseTotalForceX=off  SenseTotalForceY=off  SenseTotalForceZ=off  SenseTotalTorque=off  SenseTotalTorqueX=off  SenseTotalTorqueY=off  SenseTotalTorqueZ=off  CompositeWrenchDir=FollowerOnBase  CompositeWrenchFrame=BaseFrame
  right_wrist1 : Subsystem
  screen : Subsystem
  torso : Subsystem
  torso_t0 : sm_lib/Joints/Weld Joint  JointMode=Normal  SenseConstraintForce=off  SenseConstraintForceX=off  SenseConstraintForceY=off  SenseConstraintForceZ=off  SenseConstraintTorque=off  SenseConstraintTorqueX=off  SenseConstraintTorqueY=off  SenseConstraintTorqueZ=off  SenseTotalForce=off  SenseTotalForceX=off  SenseTotalForceY=off  SenseTotalForceZ=off  SenseTotalTorque=off  SenseTotalTorqueX=off  SenseTotalTorqueY=off  SenseTotalTorqueZ=off  CompositeWrenchDir=FollowerOnBase  CompositeWrenchFrame=BaseFrame
  q : Outport  VectorParamsAs1DForOutWhenUnconnected=off
  dq : Outport  Port=2  VectorParamsAs1DForOutWhenUnconnected=off
  torque : Outport  Port=3  VectorParamsAs1DForOutWhenUnconnected=off
  wires:
  Demux/7 -> Simulink-PS Converter6/1
  Demux/6 -> Simulink-PS Converter5/1
  Demux/2 -> Simulink-PS Converter1/1
  Demux/1 -> Simulink-PS Converter/1
  Demux/3 -> Simulink-PS Converter2/1
  Demux/5 -> Simulink-PS Converter4/1
  Demux/4 -> Simulink-PS Converter3/1
  PS-Simulink Converter10/1 -> Mux1/4
  PS-Simulink Converter5/1 -> Mux/6
  PS-Simulink Converter8/1 -> Mux1/2
  PS-Simulink Converter13/1 -> Mux1/7
  PS-Simulink Converter3/1 -> Mux/4
  PS-Simulink Converter26/1 -> Mux3/2
  PS-Simulink Converter22/1 -> Mux3/5
  PS-Simulink Converter12/1 -> Mux1/6
  PS-Simulink Converter27/1 -> Mux3/3
  Mux/1 -> Contact Force and Planar Object Motion and Visualization/4(q), q/1
  PS-Simulink Converter24/1 -> Mux3/7
  Mux1/1 -> dq/1
  PS-Simulink Converter4/1 -> Mux/5
  PS-Simulink Converter6/1 -> Mux/7
  PS-Simulink Converter7/1 -> Mux1/1
  PS-Simulink Converter11/1 -> Mux1/5
  PS-Simulink Converter23/1 -> Mux3/6
  PS-Simulink Converter25/1 -> Mux3/1
  PS-Simulink Converter/1 -> Mux/1
  PS-Simulink Converter21/1 -> Mux3/4
  PS-Simulink Converter2/1 -> Mux/3
  PS-Simulink Converter9/1 -> Mux1/3
  PS-Simulink Converter1/1 -> Mux/2
  Mux3/1 -> Subtract1/1
  [reactionTorque] -> Subtract1/2
  Subtract1/1 -> torque/1
  u/1 -> Add/1
  Add/1 -> Demux/1
  [reactionTorque] -> Add/2
  Constant/1 -> Contact Force and Planar Object Motion and Visualization/1(objectPos)
  PS-Simulink Converter29/1 -> Contact Force and Planar Object Motion and Visualization/2(endeffectorPos)
  PS-Simulink Converter30/1 -> Contact Force and Planar Object Motion and Visualization/3(endeffectorVel)
  Contact Force and Planar Object Motion and Visualization/1(reaction torque) -> [reactionTorque]
  Contact Force and Planar Object Motion and Visualization/2(reaction force) -> Scope/1
  connections:
  right_j4_2/RConn1 -- right_l4_2/LConn1
  right_j6/RConn1 -- right_l6/LConn1
  base/RConn4 -- pedestal_feet_fixed/LConn1
  right_arm_base_link/LConn1 -- right_arm_mount/RConn1
  right_wrist/RConn1 -- Transform Sensor/RConn1 -- right_wrist1/LConn1
  right_j4_2/LConn1 -- right_l4/RConn2
  pedestal/LConn1 -- pedestal_fixed/RConn1
  head_pan/LConn1 -- right_l0/RConn3
  head_camera/RConn1 -- head_camera1/LConn1
  right_j1_2/RConn1 -- right_l1_2/LConn1
  right_torso_itb/RConn1 -- right_torso_itb1/LConn1
  right_hand/LConn1 -- right_l6/RConn1
  right_arm_base_link/RConn1 -- right_j0/LConn1
  right_hand/RConn1 -- right_hand1/LConn1
  right_arm_itb/LConn1 -- right_l4/RConn3
  right_l0/RConn1 -- right_torso_itb/LConn1
  right_j1_2/LConn1 -- right_l1/RConn2
  right_j3/RConn1 -- right_l3/LConn1
  base/RConn2 -- right_arm_mount/LConn1
  head/LConn1 -- head_pan/RConn1
  right_j4/LConn1 -- right_l3/RConn1
  base/RConn1 -- torso_t0/LConn1
  right_j2_2/RConn1 -- right_l2_2/LConn1
  right_j1/RConn1 -- right_l1/LConn1
  base/RConn5 -- controller_box_fixed/LConn1
  right_hand_camera/LConn1 -- right_l5/RConn3
  right_l5/RConn1 -- right_wrist/LConn1
  pedestal_feet/LConn1 -- pedestal_feet_fixed/RConn1
  right_j1/LConn1 -- right_l0/RConn2
  display_joint/LConn1 -- head/RConn2
  right_j6/LConn1 -- right_l5/RConn2
  base/RConn3 -- pedestal_fixed/LConn1
  display_joint/RConn1 -- screen/LConn1
  right_j2_2/LConn1 -- right_l2/RConn2
  right_j5/LConn1 -- right_l4/RConn1
  right_arm_itb/RConn1 -- right_arm_itb1/LConn1
  right_j0/RConn1 -- right_l0/LConn1
  torso/LConn1 -- torso_t0/RConn1
  right_j5/RConn1 -- right_l5/LConn1
  right_hand_camera/RConn1 -- right_hand_camera1/LConn1
  right_j2/LConn1 -- right_l1/RConn1
  controller_box/LConn1 -- controller_box_fixed/RConn1
  head/RConn1 -- head_camera/LConn1
  right_j2/RConn1 -- right_l2/LConn1
  right_j4/RConn1 -- right_l4/LConn1
  right_j3/LConn1 -- right_l2/RConn1
  Simulink-PS Converter/RConn1 -- right_j0/LConn2
  Simulink-PS Converter1/RConn1 -- right_j1/LConn2
  Simulink-PS Converter2/RConn1 -- right_j2/LConn2
  Simulink-PS Converter3/RConn1 -- right_j3/LConn2
  Simulink-PS Converter4/RConn1 -- right_j4/LConn2
  Simulink-PS Converter5/RConn1 -- right_j5/LConn2
  Simulink-PS Converter6/RConn1 -- right_j6/LConn2
  right_j0/RConn2 -- PS-Simulink Converter/LConn1
  right_j1/RConn2 -- PS-Simulink Converter1/LConn1
  right_j2/RConn2 -- PS-Simulink Converter2/LConn1
  right_j3/RConn2 -- PS-Simulink Converter3/LConn1
  right_j4/RConn2 -- PS-Simulink Converter4/LConn1
  right_j5/RConn2 -- PS-Simulink Converter5/LConn1
  right_j6/RConn2 -- PS-Simulink Converter6/LConn1
  right_j0/RConn3 -- PS-Simulink Converter7/LConn1
  right_j1/RConn3 -- PS-Simulink Converter8/LConn1
  right_j2/RConn3 -- PS-Simulink Converter9/LConn1
  right_j3/RConn3 -- PS-Simulink Converter10/LConn1
  right_j4/RConn3 -- PS-Simulink Converter11/LConn1
  right_j5/RConn3 -- PS-Simulink Converter12/LConn1
  right_j6/RConn3 -- PS-Simulink Converter13/LConn1
  PS-Simulink Converter25/LConn1 -- right_j0/RConn4
  PS-Simulink Converter26/LConn1 -- right_j1/RConn4
  PS-Simulink Converter27/LConn1 -- right_j2/RConn4
  PS-Simulink Converter21/LConn1 -- right_j3/RConn4
  PS-Simulink Converter22/LConn1 -- right_j4/RConn4
  right_j5/RConn4 -- PS-Simulink Converter23/LConn1
  PS-Simulink Converter24/LConn1 -- right_j6/RConn4
  base/LConn1 -- MechanismConfiguration/RConn1 -- Contact Force and Planar Object Motion and Visualization/LConn1 -- World/RConn1 -- Solver Configuration/RConn1 -- Transform Sensor/LConn1
  Transform Sensor/RConn2 -- PS-Simulink Converter29/LConn1
  Transform Sensor/RConn3 -- PS-Simulink Converter30/LConn1

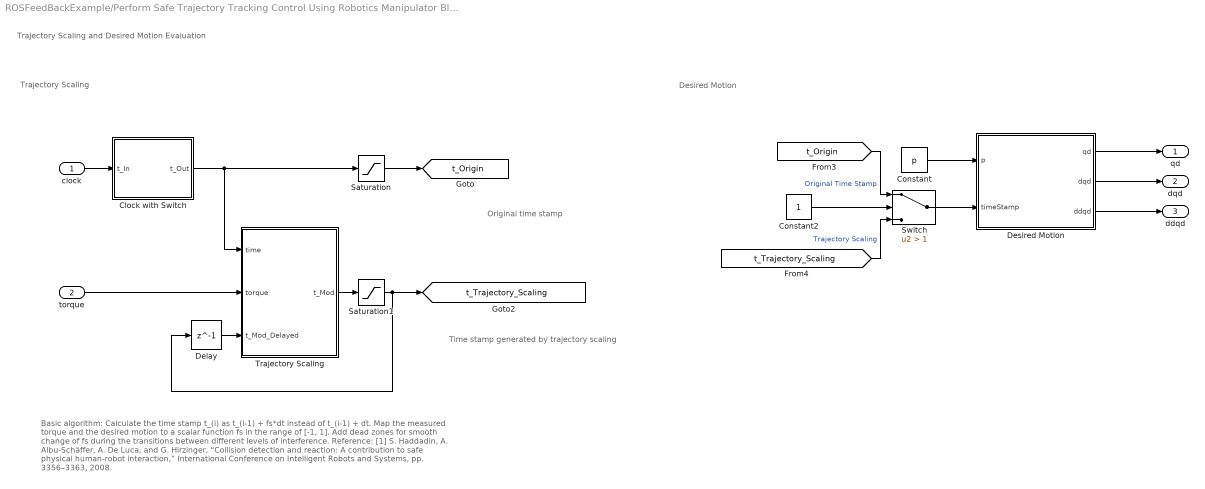
== system ROSFeedBackExample/Perform Safe Trajectory Tracking Control Using Robotics Manipulator Blocks/Trajectory Scaling and Desired Motion ==
  note: Trajectory Scaling
  note: Desired Motion
  note: Time stamp generated by trajectory scaling
  note: Original time stamp
  note: Trajectory Scaling and Desired Motion Evaluation
  note: Basic algorithm:
      | Calculate the time stamp t_(i) as t_(i-1) + fs*dt instead of t_(i-1) + dt.
      | Map the measured torque and the desired motion to a scalar function fs in the range of [-1, 1].
      | Add dead zones for smooth change of fs during the transitions between different levels of interference.
      |
      | Reference:
      | [1] S. Haddadin, A. Albu-Schäffer, A. De Luca, and G. Hirzinger, “Collision detection and reaction: A contribution to safe physical
      | human-robot interaction,” International Conference on Intelligent Robots and Systems, pp. 3356–3363, 2008.
  clock : Inport
  torque : Inport  Port=2
  Clock with Switch : Subsystem
  Constant : Constant  Value=p
  Constant2 : Constant
  Delay : Delay  DelayLength=1
  Desired Motion : MATLAB Function  TreatAsAtomicUnit=on
  Saturation : Saturate  UpperLimit=tDuration  LowerLimit=0
  Saturation1 : Saturate  UpperLimit=tDuration  LowerLimit=0
  Switch : Switch  Criteria=u2 > Threshold  Threshold=1
  Trajectory Scaling : Subsystem
  qd : Outport  VectorParamsAs1DForOutWhenUnconnected=off
  dqd : Outport  Port=2  VectorParamsAs1DForOutWhenUnconnected=off
  ddqd : Outport  Port=3  VectorParamsAs1DForOutWhenUnconnected=off
  tag scope: t_Origin=global, t_Trajectory_Scaling=global
  wires:
  Trajectory Scaling/1(t_Mod) -> Saturation1/1
  [t_Trajectory_Scaling] -> Switch/3  "Trajectory Scaling"
  Constant2/1 -> Switch/2
  Constant/1 -> Desired Motion/1(p)
  Desired Motion/1(qd) -> qd/1
  Clock with Switch/1(t_Out) -> Trajectory Scaling/1(time), Saturation/1
  Saturation/1 -> [t_Origin]
  Switch/1 -> Desired Motion/2(timeStamp)
  [t_Origin] -> Switch/1  "Original Time Stamp"
  Saturation1/1 -> Delay/1, [t_Trajectory_Scaling]
  Desired Motion/3(ddqd) -> ddqd/1
  Desired Motion/2(dqd) -> dqd/1
  clock/1 -> Clock with Switch/1(t_In)
  torque/1 -> Trajectory Scaling/2(torque)
  Delay/1 -> Trajectory Scaling/3("t_Mod_Delayed ")

== system ROSFeedBackExample/Subsystem/Check Distance To Goal ==
  robotGoal : Inport
  currentPose : Inport  Port=2
  Constant : Constant  Value=awayFromGoalThresh
  Dot Product : DotProduct  InputSameDT=on  OutDataTypeStr=Inherit: Inherit via internal rule
  Less Than : RelationalOperator  Operator=>  OutDataTypeStr=boolean  RndMeth=Simplest
  Selector : Selector  InputPortWidth=3  IndexOptions=Index vector (dialog)  Indices=[1 2]  OutputSizes=1
  Sqrt : Sqrt  SaturateOnIntegerOverflow=on
  Subtract : Sum  Inputs=+-
  atGoal : Outport
  wires:
  robotGoal/1 -> Subtract/2
  Dot Product/1 -> Sqrt/1
  Constant/1 -> Less Than/2
  currentPose/1 -> Selector/1
  Less Than/1 -> atGoal/1
  Sqrt/1 -> Less Than/1
  Subtract/1 -> Dot Product/1, Dot Product/2
  Selector/1 -> Subtract/1
